simulink model "CruiseControlSim_modified"  (R2025a)
settings: Solver=ode45  StartTime=0.0  StopTime=200  RelTol=1e-3
settings Model: Creator=Alex_  LastModifiedBy=Alex_

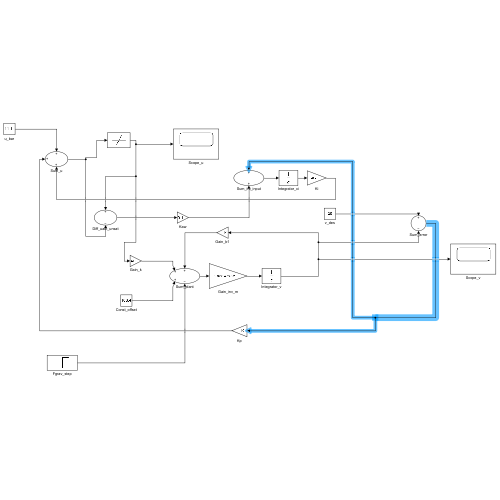
[thumbnail: Simulink's stored preview of the top-level diagram]
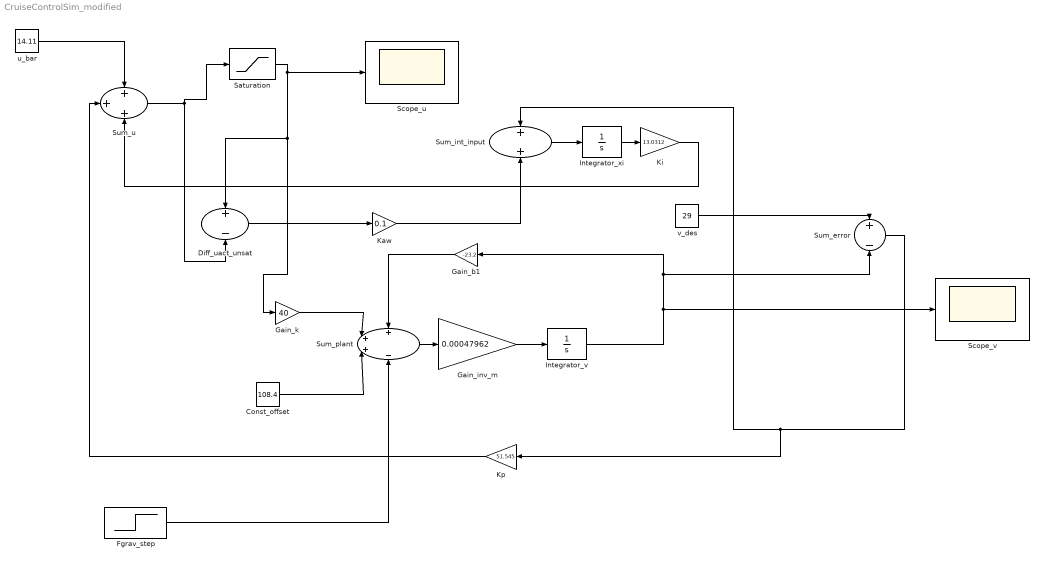
== system CruiseControlSim_modified ==
  Const_offset : Constant  Value=108.4
  Diff_uact_unsat : Sum  Inputs=+-
  Fgrav_step : Step  Time=10  After=1400  SampleTime=0
  Gain_b1 : Gain  Gain=-23.2
  Gain_inv_m : Gain  Gain=0.00047962
  Gain_k : Gain  Gain=40
  Integrator_v : Integrator  InitialCondition=29
  Integrator_xi : Integrator
  Kaw : Gain  Gain=0.1
  Ki : Gain  Gain=13.0312
  Kp : Gain  Gain=51.545
  Saturation : Saturate  UpperLimit=90  LowerLimit=0
  Scope_u : Scope
  Scope_v : Scope
  Sum_error : Sum  Inputs=+-
  Sum_int_input : Sum
  Sum_plant : Sum  Inputs=+++-
  Sum_u : Sum  Inputs=+++
  u_bar : Constant  Value=14.11
  v_des : Constant  Value=29
  wires:
  u_bar/1 -> Sum_u/1
  Fgrav_step/1 -> Sum_plant/4
  Ki/1 -> Sum_u/3
  Sum_u/1 -> Saturation/1, Diff_uact_unsat/2
  Saturation/1 -> Diff_uact_unsat/1, Gain_k/1, Scope_u/1
  Diff_uact_unsat/1 -> Kaw/1
  Const_offset/1 -> Sum_plant/3
  Sum_plant/1 -> Gain_inv_m/1
  Gain_k/1 -> Sum_plant/2
  Sum_int_input/1 -> Integrator_xi/1
  Kaw/1 -> Sum_int_input/2
  Gain_inv_m/1 -> Integrator_v/1
  Integrator_v/1 -> Gain_b1/1, Sum_error/2, Scope_v/1
  v_des/1 -> Sum_error/1
  Gain_b1/1 -> Sum_plant/1
  Sum_error/1 -> Sum_int_input/1, Kp/1
  Kp/1 -> Sum_u/2
  Integrator_xi/1 -> Ki/1
